simulink model "VACModel"  (Simulink 8.3)
settings: Solver=ode1  SolverMode=MultiTasking  StartTime=0.0  StopTime=24  FixedStep=Ts_base  MaxStep=Ts_base  MinStep=1e-6  RelTol=1e-6
PreLoadFcn:
  | initModel
StopFcn:
  | overview
undefined symbols (not defined in the file): automatic, controller_sampling_frequency, Fixed, gcr, MVs, PI, signal, transmitter_deadtime, transmitter_sampling_frequency, Ts_save, y_ss
libraries: VAlib x96
(part 17 of 18)

== system VACModel/VA Plant/xmeas atk block/xmeas3 attack controller/Attack Type Controller/periodical forward controller ==
  normal : Inport
  faked : Inport  Port=2
  Pulse Generator : DiscretePulseGenerator  PulseType=Time based  Period=duration + start  PulseWidth=100*duration/(duration + start)  PhaseDelay=start
  Switch : Switch  Criteria=u2 > Threshold
  output : Outport
  wires:
  Switch/1 -> output/1
  Pulse Generator/1 -> Switch/2
  normal/1 -> Switch/3
  faked/1 -> Switch/1

== system VACModel/VA Plant/xmeas atk block/xmeas3 attack controller/Attack Type Controller/step forward controller ==
  normal : Inport
  faked : Inport  Port=2
  Step : Step  Time=start  SampleTime=0
  Switch : Switch  Criteria=u2 > Threshold
  output : Outport
  wires:
  Switch/1 -> output/1
  Step/1 -> Switch/2
  normal/1 -> Switch/3
  faked/1 -> Switch/1

== system VACModel/VA Plant/xmeas atk block/xmeas30 attack controller/Attack Type Controller/interval forward controller ==
  normal : Inport
  faked : Inport  Port=2
  Impuls : VAlib/Impuls  amplitude=1  duration=duration  delay=start
  Switch : Switch  Criteria=u2 > Threshold
  output : Outport
  wires:
  Switch/1 -> output/1
  Impuls/1 -> Switch/2
  normal/1 -> Switch/3
  faked/1 -> Switch/1

== system VACModel/VA Plant/xmeas atk block/xmeas30 attack controller/Attack Type Controller/normal forward controller ==
  normal : Inport
  faked : Inport  Port=2
  Terminator : Terminator
  output : Outport
  wires:
  faked/1 -> Terminator/1
  normal/1 -> output/1

== system VACModel/VA Plant/xmeas atk block/xmeas30 attack controller/Attack Type Controller/periodical forward controller ==
  normal : Inport
  faked : Inport  Port=2
  Pulse Generator : DiscretePulseGenerator  PulseType=Time based  Period=duration + start  PulseWidth=100*duration/(duration + start)  PhaseDelay=start
  Switch : Switch  Criteria=u2 > Threshold
  output : Outport
  wires:
  Switch/1 -> output/1
  Pulse Generator/1 -> Switch/2
  normal/1 -> Switch/3
  faked/1 -> Switch/1

== system VACModel/VA Plant/xmeas atk block/xmeas30 attack controller/Attack Type Controller/step forward controller ==
  normal : Inport
  faked : Inport  Port=2
  Step : Step  Time=start  SampleTime=0
  Switch : Switch  Criteria=u2 > Threshold
  output : Outport
  wires:
  Switch/1 -> output/1
  Step/1 -> Switch/2
  normal/1 -> Switch/3
  faked/1 -> Switch/1

== system VACModel/VA Plant/xmeas atk block/xmeas31 attack controller/Attack Type Controller/interval forward controller ==
  normal : Inport
  faked : Inport  Port=2
  Impuls : VAlib/Impuls  amplitude=1  duration=duration  delay=start
  Switch : Switch  Criteria=u2 > Threshold
  output : Outport
  wires:
  Switch/1 -> output/1
  Impuls/1 -> Switch/2
  normal/1 -> Switch/3
  faked/1 -> Switch/1

== system VACModel/VA Plant/xmeas atk block/xmeas31 attack controller/Attack Type Controller/normal forward controller ==
  normal : Inport
  faked : Inport  Port=2
  Terminator : Terminator
  output : Outport
  wires:
  faked/1 -> Terminator/1
  normal/1 -> output/1

== system VACModel/VA Plant/xmeas atk block/xmeas31 attack controller/Attack Type Controller/periodical forward controller ==
  normal : Inport
  faked : Inport  Port=2
  Pulse Generator : DiscretePulseGenerator  PulseType=Time based  Period=duration + start  PulseWidth=100*duration/(duration + start)  PhaseDelay=start
  Switch : Switch  Criteria=u2 > Threshold
  output : Outport
  wires:
  Switch/1 -> output/1
  Pulse Generator/1 -> Switch/2
  normal/1 -> Switch/3
  faked/1 -> Switch/1

== system VACModel/VA Plant/xmeas atk block/xmeas31 attack controller/Attack Type Controller/step forward controller ==
  normal : Inport
  faked : Inport  Port=2
  Step : Step  Time=start  SampleTime=0
  Switch : Switch  Criteria=u2 > Threshold
  output : Outport
  wires:
  Switch/1 -> output/1
  Step/1 -> Switch/2
  normal/1 -> Switch/3
  faked/1 -> Switch/1

== system VACModel/VA Plant/xmeas atk block/xmeas32 attack controller/Attack Type Controller/interval forward controller ==
  normal : Inport
  faked : Inport  Port=2
  Impuls : VAlib/Impuls  amplitude=1  duration=duration  delay=start
  Switch : Switch  Criteria=u2 > Threshold
  output : Outport
  wires:
  Switch/1 -> output/1
  Impuls/1 -> Switch/2
  normal/1 -> Switch/3
  faked/1 -> Switch/1

== system VACModel/VA Plant/xmeas atk block/xmeas32 attack controller/Attack Type Controller/normal forward controller ==
  normal : Inport
  faked : Inport  Port=2
  Terminator : Terminator
  output : Outport
  wires:
  faked/1 -> Terminator/1
  normal/1 -> output/1

== system VACModel/VA Plant/xmeas atk block/xmeas32 attack controller/Attack Type Controller/periodical forward controller ==
  normal : Inport
  faked : Inport  Port=2
  Pulse Generator : DiscretePulseGenerator  PulseType=Time based  Period=duration + start  PulseWidth=100*duration/(duration + start)  PhaseDelay=start
  Switch : Switch  Criteria=u2 > Threshold
  output : Outport
  wires:
  Switch/1 -> output/1
  Pulse Generator/1 -> Switch/2
  normal/1 -> Switch/3
  faked/1 -> Switch/1

== system VACModel/VA Plant/xmeas atk block/xmeas32 attack controller/Attack Type Controller/step forward controller ==
  normal : Inport
  faked : Inport  Port=2
  Step : Step  Time=start  SampleTime=0
  Switch : Switch  Criteria=u2 > Threshold
  output : Outport
  wires:
  Switch/1 -> output/1
  Step/1 -> Switch/2
  normal/1 -> Switch/3
  faked/1 -> Switch/1

== system VACModel/VA Plant/xmeas atk block/xmeas33 attack controller/Attack Type Controller/interval forward controller ==
  normal : Inport
  faked : Inport  Port=2
  Impuls : VAlib/Impuls  amplitude=1  duration=duration  delay=start
  Switch : Switch  Criteria=u2 > Threshold
  output : Outport
  wires:
  Switch/1 -> output/1
  Impuls/1 -> Switch/2
  normal/1 -> Switch/3
  faked/1 -> Switch/1

== system VACModel/VA Plant/xmeas atk block/xmeas33 attack controller/Attack Type Controller/normal forward controller ==
  normal : Inport
  faked : Inport  Port=2
  Terminator : Terminator
  output : Outport
  wires:
  faked/1 -> Terminator/1
  normal/1 -> output/1

== system VACModel/VA Plant/xmeas atk block/xmeas33 attack controller/Attack Type Controller/periodical forward controller ==
  normal : Inport
  faked : Inport  Port=2
  Pulse Generator : DiscretePulseGenerator  PulseType=Time based  Period=duration + start  PulseWidth=100*duration/(duration + start)  PhaseDelay=start
  Switch : Switch  Criteria=u2 > Threshold
  output : Outport
  wires:
  Switch/1 -> output/1
  Pulse Generator/1 -> Switch/2
  normal/1 -> Switch/3
  faked/1 -> Switch/1

== system VACModel/VA Plant/xmeas atk block/xmeas33 attack controller/Attack Type Controller/step forward controller ==
  normal : Inport
  faked : Inport  Port=2
  Step : Step  Time=start  SampleTime=0
  Switch : Switch  Criteria=u2 > Threshold
  output : Outport
  wires:
  Switch/1 -> output/1
  Step/1 -> Switch/2
  normal/1 -> Switch/3
  faked/1 -> Switch/1

== system VACModel/VA Plant/xmeas atk block/xmeas34 attack controller/Attack Type Controller/interval forward controller ==
  normal : Inport
  faked : Inport  Port=2
  Impuls : VAlib/Impuls  amplitude=1  duration=duration  delay=start
  Switch : Switch  Criteria=u2 > Threshold
  output : Outport
  wires:
  Switch/1 -> output/1
  Impuls/1 -> Switch/2
  normal/1 -> Switch/3
  faked/1 -> Switch/1

== system VACModel/VA Plant/xmeas atk block/xmeas34 attack controller/Attack Type Controller/normal forward controller ==
  normal : Inport
  faked : Inport  Port=2
  Terminator : Terminator
  output : Outport
  wires:
  faked/1 -> Terminator/1
  normal/1 -> output/1

== system VACModel/VA Plant/xmeas atk block/xmeas34 attack controller/Attack Type Controller/periodical forward controller ==
  normal : Inport
  faked : Inport  Port=2
  Pulse Generator : DiscretePulseGenerator  PulseType=Time based  Period=duration + start  PulseWidth=100*duration/(duration + start)  PhaseDelay=start
  Switch : Switch  Criteria=u2 > Threshold
  output : Outport
  wires:
  Switch/1 -> output/1
  Pulse Generator/1 -> Switch/2
  normal/1 -> Switch/3
  faked/1 -> Switch/1

== system VACModel/VA Plant/xmeas atk block/xmeas34 attack controller/Attack Type Controller/step forward controller ==
  normal : Inport
  faked : Inport  Port=2
  Step : Step  Time=start  SampleTime=0
  Switch : Switch  Criteria=u2 > Threshold
  output : Outport
  wires:
  Switch/1 -> output/1
  Step/1 -> Switch/2
  normal/1 -> Switch/3
  faked/1 -> Switch/1

== system VACModel/VA Plant/xmeas atk block/xmeas35 attack controller/Attack Type Controller/interval forward controller ==
  normal : Inport
  faked : Inport  Port=2
  Impuls : VAlib/Impuls  amplitude=1  duration=duration  delay=start
  Switch : Switch  Criteria=u2 > Threshold
  output : Outport
  wires:
  Switch/1 -> output/1
  Impuls/1 -> Switch/2
  normal/1 -> Switch/3
  faked/1 -> Switch/1

== system VACModel/VA Plant/xmeas atk block/xmeas35 attack controller/Attack Type Controller/normal forward controller ==
  normal : Inport
  faked : Inport  Port=2
  Terminator : Terminator
  output : Outport
  wires:
  faked/1 -> Terminator/1
  normal/1 -> output/1

== system VACModel/VA Plant/xmeas atk block/xmeas35 attack controller/Attack Type Controller/periodical forward controller ==
  normal : Inport
  faked : Inport  Port=2
  Pulse Generator : DiscretePulseGenerator  PulseType=Time based  Period=duration + start  PulseWidth=100*duration/(duration + start)  PhaseDelay=start
  Switch : Switch  Criteria=u2 > Threshold
  output : Outport
  wires:
  Switch/1 -> output/1
  Pulse Generator/1 -> Switch/2
  normal/1 -> Switch/3
  faked/1 -> Switch/1

== system VACModel/VA Plant/xmeas atk block/xmeas35 attack controller/Attack Type Controller/step forward controller ==
  normal : Inport
  faked : Inport  Port=2
  Step : Step  Time=start  SampleTime=0
  Switch : Switch  Criteria=u2 > Threshold
  output : Outport
  wires:
  Switch/1 -> output/1
  Step/1 -> Switch/2
  normal/1 -> Switch/3
  faked/1 -> Switch/1

== system VACModel/VA Plant/xmeas atk block/xmeas36 attack controller/Attack Type Controller/interval forward controller ==
  normal : Inport
  faked : Inport  Port=2
  Impuls : VAlib/Impuls  amplitude=1  duration=duration  delay=start
  Switch : Switch  Criteria=u2 > Threshold
  output : Outport
  wires:
  Switch/1 -> output/1
  Impuls/1 -> Switch/2
  normal/1 -> Switch/3
  faked/1 -> Switch/1

== system VACModel/VA Plant/xmeas atk block/xmeas36 attack controller/Attack Type Controller/normal forward controller ==
  normal : Inport
  faked : Inport  Port=2
  Terminator : Terminator
  output : Outport
  wires:
  faked/1 -> Terminator/1
  normal/1 -> output/1

== system VACModel/VA Plant/xmeas atk block/xmeas36 attack controller/Attack Type Controller/periodical forward controller ==
  normal : Inport
  faked : Inport  Port=2
  Pulse Generator : DiscretePulseGenerator  PulseType=Time based  Period=duration + start  PulseWidth=100*duration/(duration + start)  PhaseDelay=start
  Switch : Switch  Criteria=u2 > Threshold
  output : Outport
  wires:
  Switch/1 -> output/1
  Pulse Generator/1 -> Switch/2
  normal/1 -> Switch/3
  faked/1 -> Switch/1

== system VACModel/VA Plant/xmeas atk block/xmeas36 attack controller/Attack Type Controller/step forward controller ==
  normal : Inport
  faked : Inport  Port=2
  Step : Step  Time=start  SampleTime=0
  Switch : Switch  Criteria=u2 > Threshold
  output : Outport
  wires:
  Switch/1 -> output/1
  Step/1 -> Switch/2
  normal/1 -> Switch/3
  faked/1 -> Switch/1

== system VACModel/VA Plant/xmeas atk block/xmeas37 attack controller/Attack Type Controller/interval forward controller ==
  normal : Inport
  faked : Inport  Port=2
  Impuls : VAlib/Impuls  amplitude=1  duration=duration  delay=start
  Switch : Switch  Criteria=u2 > Threshold
  output : Outport
  wires:
  Switch/1 -> output/1
  Impuls/1 -> Switch/2
  normal/1 -> Switch/3
  faked/1 -> Switch/1

== system VACModel/VA Plant/xmeas atk block/xmeas37 attack controller/Attack Type Controller/normal forward controller ==
  normal : Inport
  faked : Inport  Port=2
  Terminator : Terminator
  output : Outport
  wires:
  faked/1 -> Terminator/1
  normal/1 -> output/1

== system VACModel/VA Plant/xmeas atk block/xmeas37 attack controller/Attack Type Controller/periodical forward controller ==
  normal : Inport
  faked : Inport  Port=2
  Pulse Generator : DiscretePulseGenerator  PulseType=Time based  Period=duration + start  PulseWidth=100*duration/(duration + start)  PhaseDelay=start
  Switch : Switch  Criteria=u2 > Threshold
  output : Outport
  wires:
  Switch/1 -> output/1
  Pulse Generator/1 -> Switch/2
  normal/1 -> Switch/3
  faked/1 -> Switch/1

== system VACModel/VA Plant/xmeas atk block/xmeas37 attack controller/Attack Type Controller/step forward controller ==
  normal : Inport
  faked : Inport  Port=2
  Step : Step  Time=start  SampleTime=0
  Switch : Switch  Criteria=u2 > Threshold
  output : Outport
  wires:
  Switch/1 -> output/1
  Step/1 -> Switch/2
  normal/1 -> Switch/3
  faked/1 -> Switch/1

== system VACModel/VA Plant/xmeas atk block/xmeas38 attack controller/Attack Type Controller/interval forward controller ==
  normal : Inport
  faked : Inport  Port=2
  Impuls : VAlib/Impuls  amplitude=1  duration=duration  delay=start
  Switch : Switch  Criteria=u2 > Threshold
  output : Outport
  wires:
  Switch/1 -> output/1
  Impuls/1 -> Switch/2
  normal/1 -> Switch/3
  faked/1 -> Switch/1

== system VACModel/VA Plant/xmeas atk block/xmeas38 attack controller/Attack Type Controller/normal forward controller ==
  normal : Inport
  faked : Inport  Port=2
  Terminator : Terminator
  output : Outport
  wires:
  faked/1 -> Terminator/1
  normal/1 -> output/1

== system VACModel/VA Plant/xmeas atk block/xmeas38 attack controller/Attack Type Controller/periodical forward controller ==
  normal : Inport
  faked : Inport  Port=2
  Pulse Generator : DiscretePulseGenerator  PulseType=Time based  Period=duration + start  PulseWidth=100*duration/(duration + start)  PhaseDelay=start
  Switch : Switch  Criteria=u2 > Threshold
  output : Outport
  wires:
  Switch/1 -> output/1
  Pulse Generator/1 -> Switch/2
  normal/1 -> Switch/3
  faked/1 -> Switch/1

== system VACModel/VA Plant/xmeas atk block/xmeas38 attack controller/Attack Type Controller/step forward controller ==
  normal : Inport
  faked : Inport  Port=2
  Step : Step  Time=start  SampleTime=0
  Switch : Switch  Criteria=u2 > Threshold
  output : Outport
  wires:
  Switch/1 -> output/1
  Step/1 -> Switch/2
  normal/1 -> Switch/3
  faked/1 -> Switch/1

== system VACModel/VA Plant/xmeas atk block/xmeas39 attack controller/Attack Type Controller/interval forward controller ==
  normal : Inport
  faked : Inport  Port=2
  Impuls : VAlib/Impuls  amplitude=1  duration=duration  delay=start
  Switch : Switch  Criteria=u2 > Threshold
  output : Outport
  wires:
  Switch/1 -> output/1
  Impuls/1 -> Switch/2
  normal/1 -> Switch/3
  faked/1 -> Switch/1

== system VACModel/VA Plant/xmeas atk block/xmeas39 attack controller/Attack Type Controller/normal forward controller ==
  normal : Inport
  faked : Inport  Port=2
  Terminator : Terminator
  output : Outport
  wires:
  faked/1 -> Terminator/1
  normal/1 -> output/1

== system VACModel/VA Plant/xmeas atk block/xmeas39 attack controller/Attack Type Controller/periodical forward controller ==
  normal : Inport
  faked : Inport  Port=2
  Pulse Generator : DiscretePulseGenerator  PulseType=Time based  Period=duration + start  PulseWidth=100*duration/(duration + start)  PhaseDelay=start
  Switch : Switch  Criteria=u2 > Threshold
  output : Outport
  wires:
  Switch/1 -> output/1
  Pulse Generator/1 -> Switch/2
  normal/1 -> Switch/3
  faked/1 -> Switch/1

== system VACModel/VA Plant/xmeas atk block/xmeas39 attack controller/Attack Type Controller/step forward controller ==
  normal : Inport
  faked : Inport  Port=2
  Step : Step  Time=start  SampleTime=0
  Switch : Switch  Criteria=u2 > Threshold
  output : Outport
  wires:
  Switch/1 -> output/1
  Step/1 -> Switch/2
  normal/1 -> Switch/3
  faked/1 -> Switch/1

== system VACModel/VA Plant/xmeas atk block/xmeas4 attack controller/Attack Type Controller/interval forward controller ==
  normal : Inport
  faked : Inport  Port=2
  Impuls : VAlib/Impuls  amplitude=1  duration=duration  delay=start
  Switch : Switch  Criteria=u2 > Threshold
  output : Outport
  wires:
  Switch/1 -> output/1
  Impuls/1 -> Switch/2
  normal/1 -> Switch/3
  faked/1 -> Switch/1

== system VACModel/VA Plant/xmeas atk block/xmeas4 attack controller/Attack Type Controller/normal forward controller ==
  normal : Inport
  faked : Inport  Port=2
  Terminator : Terminator
  output : Outport
  wires:
  faked/1 -> Terminator/1
  normal/1 -> output/1

== system VACModel/VA Plant/xmeas atk block/xmeas4 attack controller/Attack Type Controller/periodical forward controller ==
  normal : Inport
  faked : Inport  Port=2
  Pulse Generator : DiscretePulseGenerator  PulseType=Time based  Period=duration + start  PulseWidth=100*duration/(duration + start)  PhaseDelay=start
  Switch : Switch  Criteria=u2 > Threshold
  output : Outport
  wires:
  Switch/1 -> output/1
  Pulse Generator/1 -> Switch/2
  normal/1 -> Switch/3
  faked/1 -> Switch/1

== system VACModel/VA Plant/xmeas atk block/xmeas4 attack controller/Attack Type Controller/step forward controller ==
  normal : Inport
  faked : Inport  Port=2
  Step : Step  Time=start  SampleTime=0
  Switch : Switch  Criteria=u2 > Threshold
  output : Outport
  wires:
  Switch/1 -> output/1
  Step/1 -> Switch/2
  normal/1 -> Switch/3
  faked/1 -> Switch/1

== system VACModel/VA Plant/xmeas atk block/xmeas40 attack controller/Attack Type Controller/interval forward controller ==
  normal : Inport
  faked : Inport  Port=2
  Impuls : VAlib/Impuls  amplitude=1  duration=duration  delay=start
  Switch : Switch  Criteria=u2 > Threshold
  output : Outport
  wires:
  Switch/1 -> output/1
  Impuls/1 -> Switch/2
  normal/1 -> Switch/3
  faked/1 -> Switch/1

== system VACModel/VA Plant/xmeas atk block/xmeas40 attack controller/Attack Type Controller/normal forward controller ==
  normal : Inport
  faked : Inport  Port=2
  Terminator : Terminator
  output : Outport
  wires:
  faked/1 -> Terminator/1
  normal/1 -> output/1

== system VACModel/VA Plant/xmeas atk block/xmeas40 attack controller/Attack Type Controller/periodical forward controller ==
  normal : Inport
  faked : Inport  Port=2
  Pulse Generator : DiscretePulseGenerator  PulseType=Time based  Period=duration + start  PulseWidth=100*duration/(duration + start)  PhaseDelay=start
  Switch : Switch  Criteria=u2 > Threshold
  output : Outport
  wires:
  Switch/1 -> output/1
  Pulse Generator/1 -> Switch/2
  normal/1 -> Switch/3
  faked/1 -> Switch/1

== system VACModel/VA Plant/xmeas atk block/xmeas40 attack controller/Attack Type Controller/step forward controller ==
  normal : Inport
  faked : Inport  Port=2
  Step : Step  Time=start  SampleTime=0
  Switch : Switch  Criteria=u2 > Threshold
  output : Outport
  wires:
  Switch/1 -> output/1
  Step/1 -> Switch/2
  normal/1 -> Switch/3
  faked/1 -> Switch/1

== system VACModel/VA Plant/xmeas atk block/xmeas41 attack controller/Attack Type Controller/interval forward controller ==
  normal : Inport
  faked : Inport  Port=2
  Impuls : VAlib/Impuls  amplitude=1  duration=duration  delay=start
  Switch : Switch  Criteria=u2 > Threshold
  output : Outport
  wires:
  Switch/1 -> output/1
  Impuls/1 -> Switch/2
  normal/1 -> Switch/3
  faked/1 -> Switch/1

== system VACModel/VA Plant/xmeas atk block/xmeas41 attack controller/Attack Type Controller/normal forward controller ==
  normal : Inport
  faked : Inport  Port=2
  Terminator : Terminator
  output : Outport
  wires:
  faked/1 -> Terminator/1
  normal/1 -> output/1

== system VACModel/VA Plant/xmeas atk block/xmeas41 attack controller/Attack Type Controller/periodical forward controller ==
  normal : Inport
  faked : Inport  Port=2
  Pulse Generator : DiscretePulseGenerator  PulseType=Time based  Period=duration + start  PulseWidth=100*duration/(duration + start)  PhaseDelay=start
  Switch : Switch  Criteria=u2 > Threshold
  output : Outport
  wires:
  Switch/1 -> output/1
  Pulse Generator/1 -> Switch/2
  normal/1 -> Switch/3
  faked/1 -> Switch/1

== system VACModel/VA Plant/xmeas atk block/xmeas41 attack controller/Attack Type Controller/step forward controller ==
  normal : Inport
  faked : Inport  Port=2
  Step : Step  Time=start  SampleTime=0
  Switch : Switch  Criteria=u2 > Threshold
  output : Outport
  wires:
  Switch/1 -> output/1
  Step/1 -> Switch/2
  normal/1 -> Switch/3
  faked/1 -> Switch/1

== system VACModel/VA Plant/xmeas atk block/xmeas42 attack controller/Attack Type Controller/interval forward controller ==
  normal : Inport
  faked : Inport  Port=2
  Impuls : VAlib/Impuls  amplitude=1  duration=duration  delay=start
  Switch : Switch  Criteria=u2 > Threshold
  output : Outport
  wires:
  Switch/1 -> output/1
  Impuls/1 -> Switch/2
  normal/1 -> Switch/3
  faked/1 -> Switch/1

== system VACModel/VA Plant/xmeas atk block/xmeas42 attack controller/Attack Type Controller/normal forward controller ==
  normal : Inport
  faked : Inport  Port=2
  Terminator : Terminator
  output : Outport
  wires:
  faked/1 -> Terminator/1
  normal/1 -> output/1

== system VACModel/VA Plant/xmeas atk block/xmeas42 attack controller/Attack Type Controller/periodical forward controller ==
  normal : Inport
  faked : Inport  Port=2
  Pulse Generator : DiscretePulseGenerator  PulseType=Time based  Period=duration + start  PulseWidth=100*duration/(duration + start)  PhaseDelay=start
  Switch : Switch  Criteria=u2 > Threshold
  output : Outport
  wires:
  Switch/1 -> output/1
  Pulse Generator/1 -> Switch/2
  normal/1 -> Switch/3
  faked/1 -> Switch/1

== system VACModel/VA Plant/xmeas atk block/xmeas42 attack controller/Attack Type Controller/step forward controller ==
  normal : Inport
  faked : Inport  Port=2
  Step : Step  Time=start  SampleTime=0
  Switch : Switch  Criteria=u2 > Threshold
  output : Outport
  wires:
  Switch/1 -> output/1
  Step/1 -> Switch/2
  normal/1 -> Switch/3
  faked/1 -> Switch/1

== system VACModel/VA Plant/xmeas atk block/xmeas43 attack controller/Attack Type Controller/interval forward controller ==
  normal : Inport
  faked : Inport  Port=2
  Impuls : VAlib/Impuls  amplitude=1  duration=duration  delay=start
  Switch : Switch  Criteria=u2 > Threshold
  output : Outport
  wires:
  Switch/1 -> output/1
  Impuls/1 -> Switch/2
  normal/1 -> Switch/3
  faked/1 -> Switch/1

== system VACModel/VA Plant/xmeas atk block/xmeas43 attack controller/Attack Type Controller/normal forward controller ==
  normal : Inport
  faked : Inport  Port=2
  Terminator : Terminator
  output : Outport
  wires:
  faked/1 -> Terminator/1
  normal/1 -> output/1

== system VACModel/VA Plant/xmeas atk block/xmeas43 attack controller/Attack Type Controller/periodical forward controller ==
  normal : Inport
  faked : Inport  Port=2
  Pulse Generator : DiscretePulseGenerator  PulseType=Time based  Period=duration + start  PulseWidth=100*duration/(duration + start)  PhaseDelay=start
  Switch : Switch  Criteria=u2 > Threshold
  output : Outport
  wires:
  Switch/1 -> output/1
  Pulse Generator/1 -> Switch/2
  normal/1 -> Switch/3
  faked/1 -> Switch/1

== system VACModel/VA Plant/xmeas atk block/xmeas43 attack controller/Attack Type Controller/step forward controller ==
  normal : Inport
  faked : Inport  Port=2
  Step : Step  Time=start  SampleTime=0
  Switch : Switch  Criteria=u2 > Threshold
  output : Outport
  wires:
  Switch/1 -> output/1
  Step/1 -> Switch/2
  normal/1 -> Switch/3
  faked/1 -> Switch/1

== system VACModel/VA Plant/xmeas atk block/xmeas5 attack controller/Attack Type Controller/interval forward controller ==
  normal : Inport
  faked : Inport  Port=2
  Impuls : VAlib/Impuls  amplitude=1  duration=duration  delay=start
  Switch : Switch  Criteria=u2 > Threshold
  output : Outport
  wires:
  Switch/1 -> output/1
  Impuls/1 -> Switch/2
  normal/1 -> Switch/3
  faked/1 -> Switch/1

== system VACModel/VA Plant/xmeas atk block/xmeas5 attack controller/Attack Type Controller/normal forward controller ==
  normal : Inport
  faked : Inport  Port=2
  Terminator : Terminator
  output : Outport
  wires:
  faked/1 -> Terminator/1
  normal/1 -> output/1

== system VACModel/VA Plant/xmeas atk block/xmeas5 attack controller/Attack Type Controller/periodical forward controller ==
  normal : Inport
  faked : Inport  Port=2
  Pulse Generator : DiscretePulseGenerator  PulseType=Time based  Period=duration + start  PulseWidth=100*duration/(duration + start)  PhaseDelay=start
  Switch : Switch  Criteria=u2 > Threshold
  output : Outport
  wires:
  Switch/1 -> output/1
  Pulse Generator/1 -> Switch/2
  normal/1 -> Switch/3
  faked/1 -> Switch/1

== system VACModel/VA Plant/xmeas atk block/xmeas5 attack controller/Attack Type Controller/step forward controller ==
  normal : Inport
  faked : Inport  Port=2
  Step : Step  Time=start  SampleTime=0
  Switch : Switch  Criteria=u2 > Threshold
  output : Outport
  wires:
  Switch/1 -> output/1
  Step/1 -> Switch/2
  normal/1 -> Switch/3
  faked/1 -> Switch/1

== system VACModel/VA Plant/xmeas atk block/xmeas6 attack controller/Attack Type Controller/interval forward controller ==
  normal : Inport
  faked : Inport  Port=2
  Impuls : VAlib/Impuls  amplitude=1  duration=duration  delay=start
  Switch : Switch  Criteria=u2 > Threshold
  output : Outport
  wires:
  Switch/1 -> output/1
  Impuls/1 -> Switch/2
  normal/1 -> Switch/3
  faked/1 -> Switch/1

== system VACModel/VA Plant/xmeas atk block/xmeas6 attack controller/Attack Type Controller/normal forward controller ==
  normal : Inport
  faked : Inport  Port=2
  Terminator : Terminator
  output : Outport
  wires:
  faked/1 -> Terminator/1
  normal/1 -> output/1

== system VACModel/VA Plant/xmeas atk block/xmeas6 attack controller/Attack Type Controller/periodical forward controller ==
  normal : Inport
  faked : Inport  Port=2
  Pulse Generator : DiscretePulseGenerator  PulseType=Time based  Period=duration + start  PulseWidth=100*duration/(duration + start)  PhaseDelay=start
  Switch : Switch  Criteria=u2 > Threshold
  output : Outport
  wires:
  Switch/1 -> output/1
  Pulse Generator/1 -> Switch/2
  normal/1 -> Switch/3
  faked/1 -> Switch/1

== system VACModel/VA Plant/xmeas atk block/xmeas6 attack controller/Attack Type Controller/step forward controller ==
  normal : Inport
  faked : Inport  Port=2
  Step : Step  Time=start  SampleTime=0
  Switch : Switch  Criteria=u2 > Threshold
  output : Outport
  wires:
  Switch/1 -> output/1
  Step/1 -> Switch/2
  normal/1 -> Switch/3
  faked/1 -> Switch/1

== system VACModel/VA Plant/xmeas atk block/xmeas7 attack controller/Attack Type Controller/interval forward controller ==
  normal : Inport
  faked : Inport  Port=2
  Impuls : VAlib/Impuls  amplitude=1  duration=duration  delay=start
  Switch : Switch  Criteria=u2 > Threshold
  output : Outport
  wires:
  Switch/1 -> output/1
  Impuls/1 -> Switch/2
  normal/1 -> Switch/3
  faked/1 -> Switch/1

== system VACModel/VA Plant/xmeas atk block/xmeas7 attack controller/Attack Type Controller/normal forward controller ==
  normal : Inport
  faked : Inport  Port=2
  Terminator : Terminator
  output : Outport
  wires:
  faked/1 -> Terminator/1
  normal/1 -> output/1

== system VACModel/VA Plant/xmeas atk block/xmeas7 attack controller/Attack Type Controller/periodical forward controller ==
  normal : Inport
  faked : Inport  Port=2
  Pulse Generator : DiscretePulseGenerator  PulseType=Time based  Period=duration + start  PulseWidth=100*duration/(duration + start)  PhaseDelay=start
  Switch : Switch  Criteria=u2 > Threshold
  output : Outport
  wires:
  Switch/1 -> output/1
  Pulse Generator/1 -> Switch/2
  normal/1 -> Switch/3
  faked/1 -> Switch/1

== system VACModel/VA Plant/xmeas atk block/xmeas7 attack controller/Attack Type Controller/step forward controller ==
  normal : Inport
  faked : Inport  Port=2
  Step : Step  Time=start  SampleTime=0
  Switch : Switch  Criteria=u2 > Threshold
  output : Outport
  wires:
  Switch/1 -> output/1
  Step/1 -> Switch/2
  normal/1 -> Switch/3
  faked/1 -> Switch/1

== system VACModel/VA Plant/xmeas atk block/xmeas8 attack controller/Attack Type Controller/interval forward controller ==
  normal : Inport
  faked : Inport  Port=2
  Impuls : VAlib/Impuls  amplitude=1  duration=duration  delay=start
  Switch : Switch  Criteria=u2 > Threshold
  output : Outport
  wires:
  Switch/1 -> output/1
  Impuls/1 -> Switch/2
  normal/1 -> Switch/3
  faked/1 -> Switch/1

== system VACModel/VA Plant/xmeas atk block/xmeas8 attack controller/Attack Type Controller/normal forward controller ==
  normal : Inport
  faked : Inport  Port=2
  Terminator : Terminator
  output : Outport
  wires:
  faked/1 -> Terminator/1
  normal/1 -> output/1

== system VACModel/VA Plant/xmeas atk block/xmeas8 attack controller/Attack Type Controller/periodical forward controller ==
  normal : Inport
  faked : Inport  Port=2
  Pulse Generator : DiscretePulseGenerator  PulseType=Time based  Period=duration + start  PulseWidth=100*duration/(duration + start)  PhaseDelay=start
  Switch : Switch  Criteria=u2 > Threshold
  output : Outport
  wires:
  Switch/1 -> output/1
  Pulse Generator/1 -> Switch/2
  normal/1 -> Switch/3
  faked/1 -> Switch/1

== system VACModel/VA Plant/xmeas atk block/xmeas8 attack controller/Attack Type Controller/step forward controller ==
  normal : Inport
  faked : Inport  Port=2
  Step : Step  Time=start  SampleTime=0
  Switch : Switch  Criteria=u2 > Threshold
  output : Outport
  wires:
  Switch/1 -> output/1
  Step/1 -> Switch/2
  normal/1 -> Switch/3
  faked/1 -> Switch/1

== system VACModel/VA Plant/xmeas atk block/xmeas9 attack controller/Attack Type Controller/interval forward controller ==
  normal : Inport
  faked : Inport  Port=2
  Impuls : VAlib/Impuls  amplitude=1  duration=duration  delay=start
  Switch : Switch  Criteria=u2 > Threshold
  output : Outport
  wires:
  Switch/1 -> output/1
  Impuls/1 -> Switch/2
  normal/1 -> Switch/3
  faked/1 -> Switch/1

== system VACModel/VA Plant/xmeas atk block/xmeas9 attack controller/Attack Type Controller/normal forward controller ==
  normal : Inport
  faked : Inport  Port=2
  Terminator : Terminator
  output : Outport
  wires:
  faked/1 -> Terminator/1
  normal/1 -> output/1

== system VACModel/VA Plant/xmeas atk block/xmeas9 attack controller/Attack Type Controller/periodical forward controller ==
  normal : Inport
  faked : Inport  Port=2
  Pulse Generator : DiscretePulseGenerator  PulseType=Time based  Period=duration + start  PulseWidth=100*duration/(duration + start)  PhaseDelay=start
  Switch : Switch  Criteria=u2 > Threshold
  output : Outport
  wires:
  Switch/1 -> output/1
  Pulse Generator/1 -> Switch/2
  normal/1 -> Switch/3
  faked/1 -> Switch/1

== system VACModel/VA Plant/xmeas atk block/xmeas9 attack controller/Attack Type Controller/step forward controller ==
  normal : Inport
  faked : Inport  Port=2
  Step : Step  Time=start  SampleTime=0
  Switch : Switch  Criteria=u2 > Threshold
  output : Outport
  wires:
  Switch/1 -> output/1
  Step/1 -> Switch/2
  normal/1 -> Switch/3
  faked/1 -> Switch/1

== system VACModel/VA Plant/xmv atk block/xmv1 attack controller/Attack Type Controller/interval forward controller ==
  normal : Inport
  faked : Inport  Port=2
  Impuls : VAlib/Impuls  amplitude=1  duration=duration  delay=start
  Switch : Switch  Criteria=u2 > Threshold
  output : Outport
  wires:
  Switch/1 -> output/1
  Impuls/1 -> Switch/2
  normal/1 -> Switch/3
  faked/1 -> Switch/1

== system VACModel/VA Plant/xmv atk block/xmv1 attack controller/Attack Type Controller/normal forward controller ==
  normal : Inport
  faked : Inport  Port=2
  Terminator : Terminator
  output : Outport
  wires:
  faked/1 -> Terminator/1
  normal/1 -> output/1

== system VACModel/VA Plant/xmv atk block/xmv1 attack controller/Attack Type Controller/periodical forward controller ==
  normal : Inport
  faked : Inport  Port=2
  Pulse Generator : DiscretePulseGenerator  PulseType=Time based  Period=duration + start  PulseWidth=100*duration/(duration + start)  PhaseDelay=start
  Switch : Switch  Criteria=u2 > Threshold
  output : Outport
  wires:
  Switch/1 -> output/1
  Pulse Generator/1 -> Switch/2
  normal/1 -> Switch/3
  faked/1 -> Switch/1

== system VACModel/VA Plant/xmv atk block/xmv1 attack controller/Attack Type Controller/step forward controller ==
  normal : Inport
  faked : Inport  Port=2
  Step : Step  Time=start  SampleTime=0
  Switch : Switch  Criteria=u2 > Threshold
  output : Outport
  wires:
  Switch/1 -> output/1
  Step/1 -> Switch/2
  normal/1 -> Switch/3
  faked/1 -> Switch/1

== system VACModel/VA Plant/xmv atk block/xmv10 attack controller/Attack Type Controller/interval forward controller ==
  normal : Inport
  faked : Inport  Port=2
  Impuls : VAlib/Impuls  amplitude=1  duration=duration  delay=start
  Switch : Switch  Criteria=u2 > Threshold
  output : Outport
  wires:
  Switch/1 -> output/1
  Impuls/1 -> Switch/2
  normal/1 -> Switch/3
  faked/1 -> Switch/1

== system VACModel/VA Plant/xmv atk block/xmv10 attack controller/Attack Type Controller/normal forward controller ==
  normal : Inport
  faked : Inport  Port=2
  Terminator : Terminator
  output : Outport
  wires:
  faked/1 -> Terminator/1
  normal/1 -> output/1

== system VACModel/VA Plant/xmv atk block/xmv10 attack controller/Attack Type Controller/periodical forward controller ==
  normal : Inport
  faked : Inport  Port=2
  Pulse Generator : DiscretePulseGenerator  PulseType=Time based  Period=duration + start  PulseWidth=100*duration/(duration + start)  PhaseDelay=start
  Switch : Switch  Criteria=u2 > Threshold
  output : Outport
  wires:
  Switch/1 -> output/1
  Pulse Generator/1 -> Switch/2
  normal/1 -> Switch/3
  faked/1 -> Switch/1

== system VACModel/VA Plant/xmv atk block/xmv10 attack controller/Attack Type Controller/step forward controller ==
  normal : Inport
  faked : Inport  Port=2
  Step : Step  Time=start  SampleTime=0
  Switch : Switch  Criteria=u2 > Threshold
  output : Outport
  wires:
  Switch/1 -> output/1
  Step/1 -> Switch/2
  normal/1 -> Switch/3
  faked/1 -> Switch/1

== system VACModel/VA Plant/xmv atk block/xmv11 attack controller/Attack Type Controller/interval forward controller ==
  normal : Inport
  faked : Inport  Port=2
  Impuls : VAlib/Impuls  amplitude=1  duration=duration  delay=start
  Switch : Switch  Criteria=u2 > Threshold
  output : Outport
  wires:
  Switch/1 -> output/1
  Impuls/1 -> Switch/2
  normal/1 -> Switch/3
  faked/1 -> Switch/1

== system VACModel/VA Plant/xmv atk block/xmv11 attack controller/Attack Type Controller/normal forward controller ==
  normal : Inport
  faked : Inport  Port=2
  Terminator : Terminator
  output : Outport
  wires:
  faked/1 -> Terminator/1
  normal/1 -> output/1

== system VACModel/VA Plant/xmv atk block/xmv11 attack controller/Attack Type Controller/periodical forward controller ==
  normal : Inport
  faked : Inport  Port=2
  Pulse Generator : DiscretePulseGenerator  PulseType=Time based  Period=duration + start  PulseWidth=100*duration/(duration + start)  PhaseDelay=start
  Switch : Switch  Criteria=u2 > Threshold
  output : Outport
  wires:
  Switch/1 -> output/1
  Pulse Generator/1 -> Switch/2
  normal/1 -> Switch/3
  faked/1 -> Switch/1

== system VACModel/VA Plant/xmv atk block/xmv11 attack controller/Attack Type Controller/step forward controller ==
  normal : Inport
  faked : Inport  Port=2
  Step : Step  Time=start  SampleTime=0
  Switch : Switch  Criteria=u2 > Threshold
  output : Outport
  wires:
  Switch/1 -> output/1
  Step/1 -> Switch/2
  normal/1 -> Switch/3
  faked/1 -> Switch/1

== system VACModel/VA Plant/xmv atk block/xmv12 attack controller/Attack Type Controller/interval forward controller ==
  normal : Inport
  faked : Inport  Port=2
  Impuls : VAlib/Impuls  amplitude=1  duration=duration  delay=start
  Switch : Switch  Criteria=u2 > Threshold
  output : Outport
  wires:
  Switch/1 -> output/1
  Impuls/1 -> Switch/2
  normal/1 -> Switch/3
  faked/1 -> Switch/1

== system VACModel/VA Plant/xmv atk block/xmv12 attack controller/Attack Type Controller/normal forward controller ==
  normal : Inport
  faked : Inport  Port=2
  Terminator : Terminator
  output : Outport
  wires:
  faked/1 -> Terminator/1
  normal/1 -> output/1

== system VACModel/VA Plant/xmv atk block/xmv12 attack controller/Attack Type Controller/periodical forward controller ==
  normal : Inport
  faked : Inport  Port=2
  Pulse Generator : DiscretePulseGenerator  PulseType=Time based  Period=duration + start  PulseWidth=100*duration/(duration + start)  PhaseDelay=start
  Switch : Switch  Criteria=u2 > Threshold
  output : Outport
  wires:
  Switch/1 -> output/1
  Pulse Generator/1 -> Switch/2
  normal/1 -> Switch/3
  faked/1 -> Switch/1

== system VACModel/VA Plant/xmv atk block/xmv12 attack controller/Attack Type Controller/step forward controller ==
  normal : Inport
  faked : Inport  Port=2
  Step : Step  Time=start  SampleTime=0
  Switch : Switch  Criteria=u2 > Threshold
  output : Outport
  wires:
  Switch/1 -> output/1
  Step/1 -> Switch/2
  normal/1 -> Switch/3
  faked/1 -> Switch/1

== system VACModel/VA Plant/xmv atk block/xmv13 attack controller/Attack Type Controller/interval forward controller ==
  normal : Inport
  faked : Inport  Port=2
  Impuls : VAlib/Impuls  amplitude=1  duration=duration  delay=start
  Switch : Switch  Criteria=u2 > Threshold
  output : Outport
  wires:
  Switch/1 -> output/1
  Impuls/1 -> Switch/2
  normal/1 -> Switch/3
  faked/1 -> Switch/1

== system VACModel/VA Plant/xmv atk block/xmv13 attack controller/Attack Type Controller/normal forward controller ==
  normal : Inport
  faked : Inport  Port=2
  Terminator : Terminator
  output : Outport
  wires:
  faked/1 -> Terminator/1
  normal/1 -> output/1

== system VACModel/VA Plant/xmv atk block/xmv13 attack controller/Attack Type Controller/periodical forward controller ==
  normal : Inport
  faked : Inport  Port=2
  Pulse Generator : DiscretePulseGenerator  PulseType=Time based  Period=duration + start  PulseWidth=100*duration/(duration + start)  PhaseDelay=start
  Switch : Switch  Criteria=u2 > Threshold
  output : Outport
  wires:
  Switch/1 -> output/1
  Pulse Generator/1 -> Switch/2
  normal/1 -> Switch/3
  faked/1 -> Switch/1

== system VACModel/VA Plant/xmv atk block/xmv13 attack controller/Attack Type Controller/step forward controller ==
  normal : Inport
  faked : Inport  Port=2
  Step : Step  Time=start  SampleTime=0
  Switch : Switch  Criteria=u2 > Threshold
  output : Outport
  wires:
  Switch/1 -> output/1
  Step/1 -> Switch/2
  normal/1 -> Switch/3
  faked/1 -> Switch/1

== system VACModel/VA Plant/xmv atk block/xmv14 attack controller/Attack Type Controller/interval forward controller ==
  normal : Inport
  faked : Inport  Port=2
  Impuls : VAlib/Impuls  amplitude=1  duration=duration  delay=start
  Switch : Switch  Criteria=u2 > Threshold
  output : Outport
  wires:
  Switch/1 -> output/1
  Impuls/1 -> Switch/2
  normal/1 -> Switch/3
  faked/1 -> Switch/1

== system VACModel/VA Plant/xmv atk block/xmv14 attack controller/Attack Type Controller/normal forward controller ==
  normal : Inport
  faked : Inport  Port=2
  Terminator : Terminator
  output : Outport
  wires:
  faked/1 -> Terminator/1
  normal/1 -> output/1

== system VACModel/VA Plant/xmv atk block/xmv14 attack controller/Attack Type Controller/periodical forward controller ==
  normal : Inport
  faked : Inport  Port=2
  Pulse Generator : DiscretePulseGenerator  PulseType=Time based  Period=duration + start  PulseWidth=100*duration/(duration + start)  PhaseDelay=start
  Switch : Switch  Criteria=u2 > Threshold
  output : Outport
  wires:
  Switch/1 -> output/1
  Pulse Generator/1 -> Switch/2
  normal/1 -> Switch/3
  faked/1 -> Switch/1

== system VACModel/VA Plant/xmv atk block/xmv14 attack controller/Attack Type Controller/step forward controller ==
  normal : Inport
  faked : Inport  Port=2
  Step : Step  Time=start  SampleTime=0
  Switch : Switch  Criteria=u2 > Threshold
  output : Outport
  wires:
  Switch/1 -> output/1
  Step/1 -> Switch/2
  normal/1 -> Switch/3
  faked/1 -> Switch/1

== system VACModel/VA Plant/xmv atk block/xmv15 attack controller/Attack Type Controller/interval forward controller ==
  normal : Inport
  faked : Inport  Port=2
  Impuls : VAlib/Impuls  amplitude=1  duration=duration  delay=start
  Switch : Switch  Criteria=u2 > Threshold
  output : Outport
  wires:
  Switch/1 -> output/1
  Impuls/1 -> Switch/2
  normal/1 -> Switch/3
  faked/1 -> Switch/1

== system VACModel/VA Plant/xmv atk block/xmv15 attack controller/Attack Type Controller/normal forward controller ==
  normal : Inport
  faked : Inport  Port=2
  Terminator : Terminator
  output : Outport
  wires:
  faked/1 -> Terminator/1
  normal/1 -> output/1

== system VACModel/VA Plant/xmv atk block/xmv15 attack controller/Attack Type Controller/periodical forward controller ==
  normal : Inport
  faked : Inport  Port=2
  Pulse Generator : DiscretePulseGenerator  PulseType=Time based  Period=duration + start  PulseWidth=100*duration/(duration + start)  PhaseDelay=start
  Switch : Switch  Criteria=u2 > Threshold
  output : Outport
  wires:
  Switch/1 -> output/1
  Pulse Generator/1 -> Switch/2
  normal/1 -> Switch/3
  faked/1 -> Switch/1

== system VACModel/VA Plant/xmv atk block/xmv15 attack controller/Attack Type Controller/step forward controller ==
  normal : Inport
  faked : Inport  Port=2
  Step : Step  Time=start  SampleTime=0
  Switch : Switch  Criteria=u2 > Threshold
  output : Outport
  wires:
  Switch/1 -> output/1
  Step/1 -> Switch/2
  normal/1 -> Switch/3
  faked/1 -> Switch/1

== system VACModel/VA Plant/xmv atk block/xmv16 attack controller/Attack Type Controller/interval forward controller ==
  normal : Inport
  faked : Inport  Port=2
  Impuls : VAlib/Impuls  amplitude=1  duration=duration  delay=start
  Switch : Switch  Criteria=u2 > Threshold
  output : Outport
  wires:
  Switch/1 -> output/1
  Impuls/1 -> Switch/2
  normal/1 -> Switch/3
  faked/1 -> Switch/1

== system VACModel/VA Plant/xmv atk block/xmv16 attack controller/Attack Type Controller/normal forward controller ==
  normal : Inport
  faked : Inport  Port=2
  Terminator : Terminator
  output : Outport
  wires:
  faked/1 -> Terminator/1
  normal/1 -> output/1

== system VACModel/VA Plant/xmv atk block/xmv16 attack controller/Attack Type Controller/periodical forward controller ==
  normal : Inport
  faked : Inport  Port=2
  Pulse Generator : DiscretePulseGenerator  PulseType=Time based  Period=duration + start  PulseWidth=100*duration/(duration + start)  PhaseDelay=start
  Switch : Switch  Criteria=u2 > Threshold
  output : Outport
  wires:
  Switch/1 -> output/1
  Pulse Generator/1 -> Switch/2
  normal/1 -> Switch/3
  faked/1 -> Switch/1

== system VACModel/VA Plant/xmv atk block/xmv16 attack controller/Attack Type Controller/step forward controller ==
  normal : Inport
  faked : Inport  Port=2
  Step : Step  Time=start  SampleTime=0
  Switch : Switch  Criteria=u2 > Threshold
  output : Outport
  wires:
  Switch/1 -> output/1
  Step/1 -> Switch/2
  normal/1 -> Switch/3
  faked/1 -> Switch/1

== system VACModel/VA Plant/xmv atk block/xmv17 attack controller/Attack Type Controller/interval forward controller ==
  normal : Inport
  faked : Inport  Port=2
  Impuls : VAlib/Impuls  amplitude=1  duration=duration  delay=start
  Switch : Switch  Criteria=u2 > Threshold
  output : Outport
  wires:
  Switch/1 -> output/1
  Impuls/1 -> Switch/2
  normal/1 -> Switch/3
  faked/1 -> Switch/1

== system VACModel/VA Plant/xmv atk block/xmv17 attack controller/Attack Type Controller/normal forward controller ==
  normal : Inport
  faked : Inport  Port=2
  Terminator : Terminator
  output : Outport
  wires:
  faked/1 -> Terminator/1
  normal/1 -> output/1

== system VACModel/VA Plant/xmv atk block/xmv17 attack controller/Attack Type Controller/periodical forward controller ==
  normal : Inport
  faked : Inport  Port=2
  Pulse Generator : DiscretePulseGenerator  PulseType=Time based  Period=duration + start  PulseWidth=100*duration/(duration + start)  PhaseDelay=start
  Switch : Switch  Criteria=u2 > Threshold
  output : Outport
  wires:
  Switch/1 -> output/1
  Pulse Generator/1 -> Switch/2
  normal/1 -> Switch/3
  faked/1 -> Switch/1

== system VACModel/VA Plant/xmv atk block/xmv17 attack controller/Attack Type Controller/step forward controller ==
  normal : Inport
  faked : Inport  Port=2
  Step : Step  Time=start  SampleTime=0
  Switch : Switch  Criteria=u2 > Threshold
  output : Outport
  wires:
  Switch/1 -> output/1
  Step/1 -> Switch/2
  normal/1 -> Switch/3
  faked/1 -> Switch/1

== system VACModel/VA Plant/xmv atk block/xmv18 attack controller/Attack Type Controller/interval forward controller ==
  normal : Inport
  faked : Inport  Port=2
  Impuls : VAlib/Impuls  amplitude=1  duration=duration  delay=start
  Switch : Switch  Criteria=u2 > Threshold
  output : Outport
  wires:
  Switch/1 -> output/1
  Impuls/1 -> Switch/2
  normal/1 -> Switch/3
  faked/1 -> Switch/1

== system VACModel/VA Plant/xmv atk block/xmv18 attack controller/Attack Type Controller/normal forward controller ==
  normal : Inport
  faked : Inport  Port=2
  Terminator : Terminator
  output : Outport
  wires:
  faked/1 -> Terminator/1
  normal/1 -> output/1

== system VACModel/VA Plant/xmv atk block/xmv18 attack controller/Attack Type Controller/periodical forward controller ==
  normal : Inport
  faked : Inport  Port=2
  Pulse Generator : DiscretePulseGenerator  PulseType=Time based  Period=duration + start  PulseWidth=100*duration/(duration + start)  PhaseDelay=start
  Switch : Switch  Criteria=u2 > Threshold
  output : Outport
  wires:
  Switch/1 -> output/1
  Pulse Generator/1 -> Switch/2
  normal/1 -> Switch/3
  faked/1 -> Switch/1

== system VACModel/VA Plant/xmv atk block/xmv18 attack controller/Attack Type Controller/step forward controller ==
  normal : Inport
  faked : Inport  Port=2
  Step : Step  Time=start  SampleTime=0
  Switch : Switch  Criteria=u2 > Threshold
  output : Outport
  wires:
  Switch/1 -> output/1
  Step/1 -> Switch/2
  normal/1 -> Switch/3
  faked/1 -> Switch/1

== system VACModel/VA Plant/xmv atk block/xmv19 attack controller/Attack Type Controller/interval forward controller ==
  normal : Inport
  faked : Inport  Port=2
  Impuls : VAlib/Impuls  amplitude=1  duration=duration  delay=start
  Switch : Switch  Criteria=u2 > Threshold
  output : Outport
  wires:
  Switch/1 -> output/1
  Impuls/1 -> Switch/2
  normal/1 -> Switch/3
  faked/1 -> Switch/1

== system VACModel/VA Plant/xmv atk block/xmv19 attack controller/Attack Type Controller/normal forward controller ==
  normal : Inport
  faked : Inport  Port=2
  Terminator : Terminator
  output : Outport
  wires:
  faked/1 -> Terminator/1
  normal/1 -> output/1

== system VACModel/VA Plant/xmv atk block/xmv19 attack controller/Attack Type Controller/periodical forward controller ==
  normal : Inport
  faked : Inport  Port=2
  Pulse Generator : DiscretePulseGenerator  PulseType=Time based  Period=duration + start  PulseWidth=100*duration/(duration + start)  PhaseDelay=start
  Switch : Switch  Criteria=u2 > Threshold
  output : Outport
  wires:
  Switch/1 -> output/1
  Pulse Generator/1 -> Switch/2
  normal/1 -> Switch/3
  faked/1 -> Switch/1

== system VACModel/VA Plant/xmv atk block/xmv19 attack controller/Attack Type Controller/step forward controller ==
  normal : Inport
  faked : Inport  Port=2
  Step : Step  Time=start  SampleTime=0
  Switch : Switch  Criteria=u2 > Threshold
  output : Outport
  wires:
  Switch/1 -> output/1
  Step/1 -> Switch/2
  normal/1 -> Switch/3
  faked/1 -> Switch/1

== system VACModel/VA Plant/xmv atk block/xmv2 attack controller/Attack Type Controller/interval forward controller ==
  normal : Inport
  faked : Inport  Port=2
  Impuls : VAlib/Impuls  amplitude=1  duration=duration  delay=start
  Switch : Switch  Criteria=u2 > Threshold
  output : Outport
  wires:
  Switch/1 -> output/1
  Impuls/1 -> Switch/2
  normal/1 -> Switch/3
  faked/1 -> Switch/1

== system VACModel/VA Plant/xmv atk block/xmv2 attack controller/Attack Type Controller/normal forward controller ==
  normal : Inport
  faked : Inport  Port=2
  Terminator : Terminator
  output : Outport
  wires:
  faked/1 -> Terminator/1
  normal/1 -> output/1

== system VACModel/VA Plant/xmv atk block/xmv2 attack controller/Attack Type Controller/periodical forward controller ==
  normal : Inport
  faked : Inport  Port=2
  Pulse Generator : DiscretePulseGenerator  PulseType=Time based  Period=duration + start  PulseWidth=100*duration/(duration + start)  PhaseDelay=start
  Switch : Switch  Criteria=u2 > Threshold
  output : Outport
  wires:
  Switch/1 -> output/1
  Pulse Generator/1 -> Switch/2
  normal/1 -> Switch/3
  faked/1 -> Switch/1

== system VACModel/VA Plant/xmv atk block/xmv2 attack controller/Attack Type Controller/step forward controller ==
  normal : Inport
  faked : Inport  Port=2
  Step : Step  Time=start  SampleTime=0
  Switch : Switch  Criteria=u2 > Threshold
  output : Outport
  wires:
  Switch/1 -> output/1
  Step/1 -> Switch/2
  normal/1 -> Switch/3
  faked/1 -> Switch/1
